simulink model "model_nabl"  (R2024a)
settings: Solver=VariableStepAuto  StartTime=0.0  StopTime=10.0  RelTol=1e-3
settings Model: Creator=eva  LastModifiedBy=eva

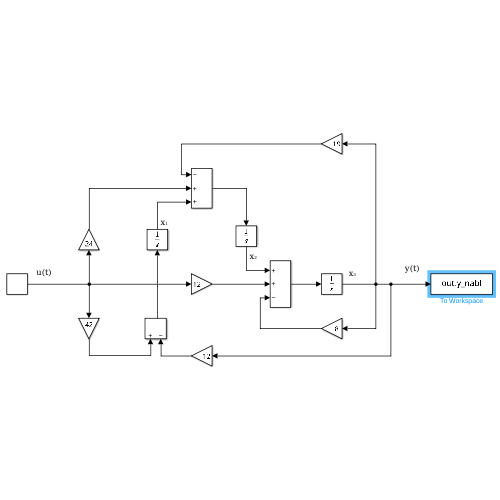
[thumbnail: Simulink's stored preview of the top-level diagram]
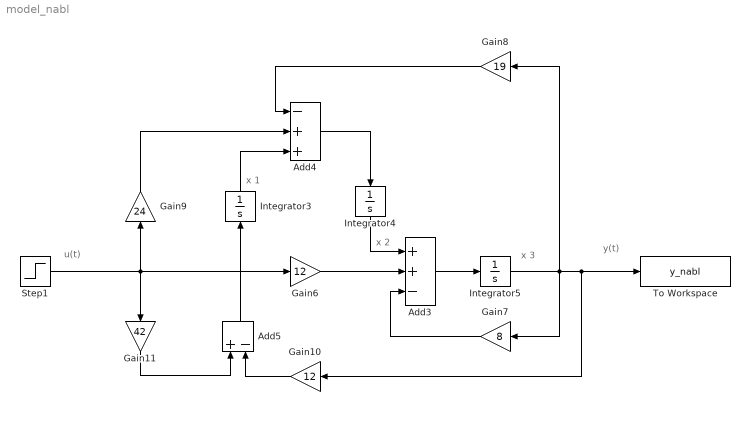
== system model_nabl ==
  note: u(t)
  note: x 3
  note: y(t)
  note: x 2
  note: x 1
  Add3 : Sum  Inputs=++-
  Add4 : Sum  Inputs=-++
  Add5 : Sum  Inputs=+-
  Gain10 : Gain  Gain=12
  Gain11 : Gain  Gain=42
  Gain6 : Gain  Gain=12
  Gain7 : Gain  Gain=8
  Gain8 : Gain  Gain=19
  Gain9 : Gain  Gain=24
  Integrator3 : Integrator
  Integrator4 : Integrator
  Integrator5 : Integrator
  Step1 : Step  Time=0  SampleTime=0
  To Workspace : ToWorkspace  VariableName=y_nabl  SaveFormat=Structure With Time  SampleTime=-1
  wires:
  Integrator5/1 -> To Workspace/1, Gain10/1, Gain7/1, Gain8/1
  Gain7/1 -> Add3/3
  Gain6/1 -> Add3/2
  Add3/1 -> Integrator5/1
  Gain10/1 -> Add5/2
  Add5/1 -> Integrator3/1
  Integrator4/1 -> Add3/1
  Step1/1 -> Gain11/1, Gain6/1, Gain9/1
  Add4/1 -> Integrator4/1
  Gain9/1 -> Add4/2
  Gain8/1 -> Add4/1
  Gain11/1 -> Add5/1
  Integrator3/1 -> Add4/3
